simulink model "fco"  (R2020b)
settings: Solver=VariableStepAuto  StartTime=0.0  StopTime=2500  RelTol=1e-3
undefined symbols (not defined in the file): a0, a1, a2, b0, b1, b2, d
settings Model: Creator=danes  LastModifiedBy=danes

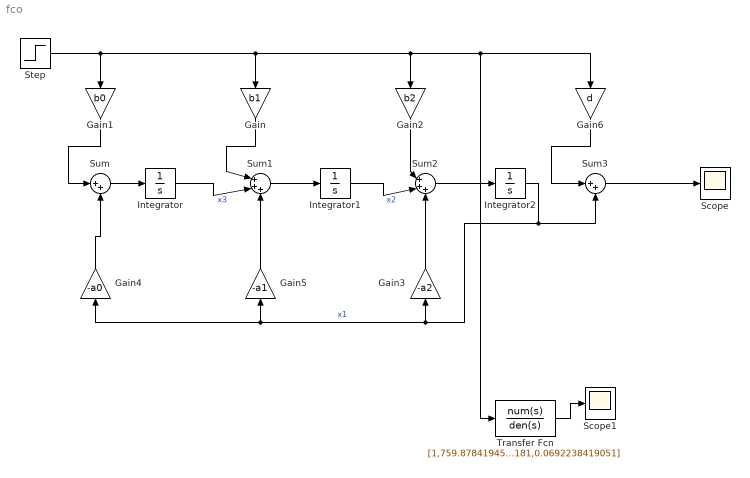
== system fco ==
  Gain : Gain  Gain=b1
  Gain1 : Gain  Gain=b0
  Gain2 : Gain  Gain=b2
  Gain3 : Gain  Gain=-a2
  Gain4 : Gain  Gain=-a0
  Gain5 : Gain  Gain=-a1
  Gain6 : Gain  Gain=d
  Integrator : Integrator
  Integrator1 : Integrator
  Integrator2 : Integrator
  Scope : Scope
  Scope1 : Scope
  Step : Step  SampleTime=0
  Sum : Sum  Inputs=|++
  Sum1 : Sum  Inputs=|+++
  Sum2 : Sum  Inputs=|+++
  Sum3 : Sum  Inputs=|++
  Transfer Fcn : TransferFcn  Numerator=[1,759.8784194528876,41.1189620916066,0.0692238419051]  Denominator=[1,759.8817864562545,43.6774752884181,0.0692238419051]
  wires:
  Step/1 -> Transfer Fcn/1, Gain6/1, Gain2/1, Gain/1, Gain1/1
  Gain6/1 -> Sum3/1
  Integrator2/1 -> Gain4/1, Gain5/1, Gain3/1, Sum3/2  "x1"
  Sum2/1 -> Integrator2/1
  Gain2/1 -> Sum2/1
  Gain3/1 -> Sum2/3
  Integrator1/1 -> Sum2/2  "x2"
  Sum1/1 -> Integrator1/1
  Gain/1 -> Sum1/1
  Gain5/1 -> Sum1/3
  Integrator/1 -> Sum1/2  "x3"
  Gain4/1 -> Sum/2
  Sum/1 -> Integrator/1
  Gain1/1 -> Sum/1
  Sum3/1 -> Scope/1
  Transfer Fcn/1 -> Scope1/1
